simulink model "LQR"  (R2020a)
settings: Solver=FixedStepAuto  StartTime=0.0  StopTime=20  FixedStep=Ts  RelTol=1e-3
values from neighbouring files (symbols this model uses):
  down = -up    (= -0.0872664625997)    [LQR.m]
  K1 = 6.1486    [LQR.m]
  up = 5*pi/180    (= 0.0872664625997)    [LQR.m]
undefined symbols (not defined in the file or in its folder): A, B, C
libraries: simulink x4
settings Model: Creator=Ashraf  LastModifiedBy=hhiastt
settings DataIOCC: ReturnWorkspaceOutputs=off
settings DebuggingCC: ArithmeticOperatorsInVariantConditions=warning
settings SFSimCC: SimUseLocalCustomCode=off  CustomCodeUndefinedFunction=UseInterfaceOnly
settings RTWCC: RTWUseLocalCustomCode=off
settings CodeAppCC: StateflowObjectComments=on

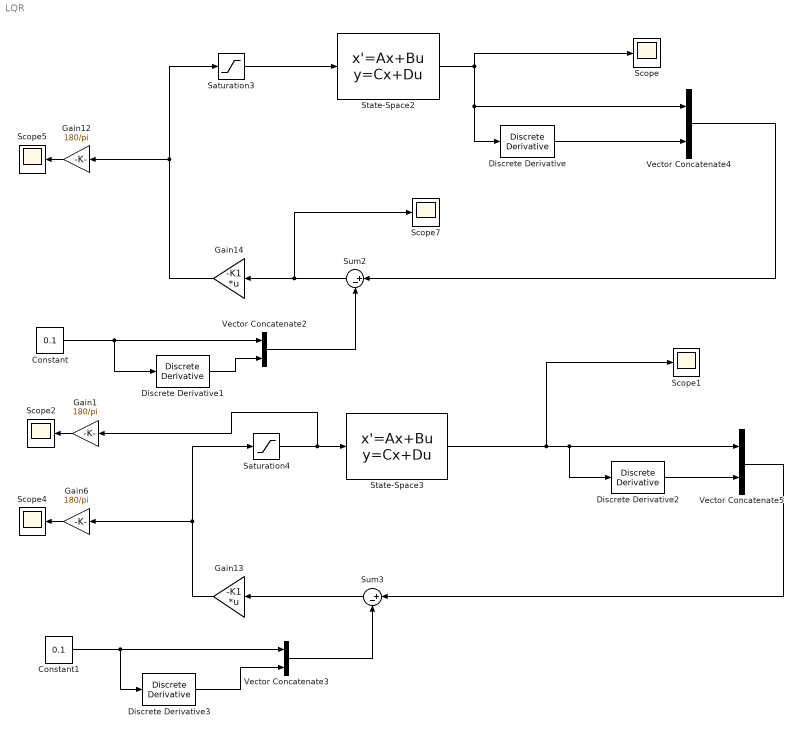
== system LQR ==
  Constant : Constant  Value=0.1
  Constant1 : Constant  Value=0.1
  Discrete Derivative{,1..3} (4 alike) : simulink/Discrete/Discrete Derivative  gainval=1.0  ICPrevScaledInput=0.0  OutMin=[]  OutMax=[]  OutDataType=fixdt(1, 16)  OutScaling=2^-10  DoSatur=off
  Gain1 : Gain  Gain=180/pi
  Gain12 : Gain  Gain=180/pi
  Gain13 : Gain  Gain=-K1  Multiplication=Matrix(K*u)
  Gain14 : Gain  Gain=-K1  Multiplication=Matrix(K*u)
  Gain6 : Gain  Gain=180/pi
  Saturation3 : Saturate  UpperLimit=up  LowerLimit=down  ZeroCross=off
  Saturation4 : Saturate  UpperLimit=up  LowerLimit=down  ZeroCross=off
  Scope{,1..2,4..5,7} (6 alike) : Scope
  State-Space2 : StateSpace  A=A  B=B  C=C  D=0  InitialCondition=[0 0]
  State-Space3 : StateSpace  A=A  B=B  C=C  D=0  InitialCondition=[0 0]
  Sum2 : Sum  Inputs=|+-
  Sum3 : Sum  Inputs=|+-
  Vector Concatenate{2..5} (4 alike) : Concatenate
  wires:
  Vector Concatenate3/1 -> Sum3/2
  Sum3/1 -> Gain13/1
  Constant1/1 -> Discrete Derivative3/1, Vector Concatenate3/1
  Constant/1 -> Discrete Derivative1/1, Vector Concatenate2/1
  Gain13/1 -> Gain6/1, Saturation4/1
  Gain14/1 -> Saturation3/1, Gain12/1
  Vector Concatenate2/1 -> Sum2/2
  State-Space3/1 -> Scope1/1, Discrete Derivative2/1, Vector Concatenate5/1
  Sum2/1 -> Scope7/1, Gain14/1
  Gain6/1 -> Scope4/1
  Gain12/1 -> Scope5/1
  Discrete Derivative3/1 -> Vector Concatenate3/2
  Discrete Derivative/1 -> Vector Concatenate4/2
  Discrete Derivative2/1 -> Vector Concatenate5/2
  Vector Concatenate4/1 -> Sum2/1
  Discrete Derivative1/1 -> Vector Concatenate2/2
  Vector Concatenate5/1 -> Sum3/1
  State-Space2/1 -> Scope/1, Vector Concatenate4/1, Discrete Derivative/1
  Saturation3/1 -> State-Space2/1
  Gain1/1 -> Scope2/1
  Saturation4/1 -> Gain1/1, State-Space3/1
